simulink model "UnusedModels"  (R2015a)
settings: Solver=ode45  StartTime=0.0  StopTime=10.0  RelTol=1e-3
values from neighbouring files (symbols this model uses):
  car_params = Simulink_Car_params    [TV2016_parameters.m]
  energyLimitControl = Simulink_energyLimit    [TV2016_parameters.m]
  settings = Simulink_Settings    [TV2016_parameters.m]
  speedEstimation = Simulink_speedEst    [TV2016_parameters.m]
  tractionControl = Simulink_tc    [TV2016_parameters.m]
  yawRateControl = Simulink_yawRate    [TV2016_parameters.m]
undefined symbols (not defined in the file or in its folder): canChannel, Use_Estimated_velocity
libraries: canlib x44, CarMaker4SL x33, canmsglib x28, simulink x6
(part 3 of 4)

== matlab function UnusedModels/speedEstimate/Vestimate ==
  data: sensors input; V_est_x output; whl_speed output Bus: Whl_speed; Y_meas output; front_rear_Var output; front_Var output; rear_Var output; all_Var output; left_Var output; right_Var output; RPM_derivative input Bus: RPMDerivative; normalForces input Bus: normalForces; settings parameter; car_params parameter; speedEstimation parameter
function [V_est_x,whl_speed, Y_meas,front_rear_Var,front_Var,rear_Var,all_Var,left_Var,right_Var]...
         = SpeedEstimations(sensors,RPM_derivative,normalForces,settings,car_params,speedEstimation)
     
     
     %rateRPM_FL, rateRPM_FR,rateRPM_RL,rateRPM_RR,sensor,settings,car_params)
%#codegen

% ------------------------------
% DECLARATIONS
% ------------------------------
persistent firstIteration;
persistent v;
persistent error;
persistent K;
k_FL = single(0); % Gain 
k_FR = single(0); % Gain
k_RL = single(0); % Gain
k_RR = single(0); % Gain
% Gains for trusting, not trusting wheel speed measurements
Hg = speedEstimation.High_gain;
Lg = speedEstimation.Low_gain;
% Variances
all_Var = single(0); % Variance for all measurements
front_rear_Var = single(0);
front_Var = single(0);
rear_Var = single(0);
left_Var = single(0);
right_Var = single(0);
% LIMITS:
velocity_deviation_limit = speedEstimation.velocity_deviation_limit;
lim = speedEstimation.variance_limit;
RPM_derivative_limit = speedEstimation.RPM_derivative_limit;

% Measurement vector
C = [1;1;1;1]; % Create four copies of predicted vx

pikk = int32(50);
% ------------------------------
% PARAMETERS
% ------------------------------
%Conversion from RPM to rad/s for the wheel
c = single(2*pi/(car_params.GR*60));
t = settings.control_system_sample_time;
%Weights taken from wikipedia
%sg_Weight = single( [ 1; -8; 0; 8; -1] );
sg_Weight = single( [ -1; 8; 0; -8; 1] );
%sg_Weight = single([0.3; 0.1; -0.1 ; -0.3]);
%sg_Weight = single([1; -1; 0 ; -0]);
% ------------------------------
% COPY VARIABLES EACH TIMESTEP
% ------------------------------
S = sensors.Input_steering; % Steering angle in rad( Mean of front wheels)
ax = sensors.ax; % Should be true linear acceleration compensated for roll angle
%Fz, used to determine what wheel speeds to trust.
Fz = [normalForces.FL, normalForces.FR, normalForces.RL ,normalForces.RR];
% Determine CoG Vx from motor RPM. Simple atm. Not considering vy.
Whl_v_FL = sensors.RPM_FL*c*car_params.r_eff*cos(S) + sensors.r*car_params.t_f;
Whl_v_FR = sensors.RPM_FR*c*car_params.r_eff*cos(S) - sensors.r*car_params.t_f;
Whl_v_RL = sensors.RPM_RL*c*car_params.r_eff + sensors.r*car_params.t_r;
Whl_v_RR = sensors.RPM_RR*c*car_params.r_eff - sensors.r*car_params.t_r;
whl_speed.v_FL = Whl_v_FL;
whl_speed.v_FR = Whl_v_FR;
whl_speed.v_RL = Whl_v_RL;
whl_speed.v_RR = Whl_v_RR;


RPM = [sensors.RPM_FL, sensors.RPM_FR, sensors.RPM_RL, sensors.RPM_RR]';
% Measurement vector, compensated RPMS
Y_meas = [Whl_v_FL, Whl_v_FR, Whl_v_RL, Whl_v_RR]';
% Input Derivative of RPM
rateRPM_FL = RPM_derivative.FL;
rateRPM_FR = RPM_derivative.FR;
rateRPM_RL = RPM_derivative.RL;
rateRPM_RR = RPM_derivative.RR;

% Different sums of normal forces, used to determine what wheels to trust
left_Fz = sum(Fz([1 3]));
right_Fz = sum(Fz([2 4]));
front_Fz = sum(Fz(1:2));
rear_Fz = sum(Fz(3:4));

% ------------------------------
% ESTIMATE DERIVATIVE OF COMPENSATED MOTOR RPM
% ------------------------------
% Problem with noise from yaw rate coupling into the derivative.. 
% Can I use uncompensated front wheels ? Should not be slipping like crazy
% with a significant steering angle ? 

% First try is with pure RPMS
% rateRPM_FL = simpleNumericalDerivative_RPM(sensor.RPM_FL,t);
% rateRPM_FR = simpleNumericalDerivative_RPM(sensor.RPM_FR,t);
% rateRPM_RL = simpleNumericalDerivative_RPM(sensor.RPM_RL,t);
% rateRPM_RR = simpleNumericalDerivative_RPM(sensor.RPM_RR,t);


% ------------------------------
% DRIFTING INS VELOCITY
% ------------------------------
persistent drift;




% ALGORITHM
if isempty(firstIteration)
    K = single(ones(1,4));
    v = single(0);
    V_est_x = v;
    error = Y_meas- C*v;
    firstIteration = 2;
    drift = single(0);
else
    drift = drift + 0.03*t;
    v_ins = sensors.V_x + 0.05 + drift;
    v = v + t*ax;
    %v = v + t*(ax + K*error);
    error = Y_meas - C*v ;
    V_est_x = 0.98*v;
    
    % Find K
    % Divide by zero problems...
    mean_WhlV = max(0.001,mean(Y_meas));
    mean_front_WhlV = max(0.001,mean(Y_meas(1:2)));
    mean_rear_WhlV  = max(0.001,mean(Y_meas(3:4)));
    mean_left_WhlV  = max(0.001,mean(Y_meas([1 3])));
    mean_right_WhlV = max(0.001,mean(Y_meas([2 4])));

    all_Var = var(Y_meas,1)/mean_WhlV;
    front_rear_Var = var([mean_front_WhlV, mean_rear_WhlV],1)/mean_WhlV;
    front_Var = var(Y_meas(1:2),1)/mean_front_WhlV;
    rear_Var  = var(Y_meas(3:4),1)/mean_rear_WhlV;
    
    left_Var    = var(Y_meas([1 3]),1)/mean_left_WhlV;
    right_Var   = var(Y_meas([2 4]),1)/mean_right_WhlV;   
    
    if (  (abs(Whl_v_FL - v_ins) > velocity_deviation_limit)...
       && (abs(Whl_v_FR - v_ins) > velocity_deviation_limit)...
       && (abs(Whl_v_RL - v_ins) > velocity_deviation_limit)...
       && (abs(Whl_v_RR - v_ins) > velocity_deviation_limit) )
        
        K = [Lg, Lg, Lg, Lg];
    
    elseif (all_Var  < lim ) 
        % low variance for all wheels.
        % Check derivative of motor RPM
        if ( (rateRPM_FL > RPM_derivative_limit) ||...
             (rateRPM_FR > RPM_derivative_limit) ||...
             (rateRPM_RL > RPM_derivative_limit) ||...
             (rateRPM_RR > RPM_derivative_limit))
            K = [Lg, Lg, Lg, Lg];
        % Rate of change of RPM can be low but slip rate is large
        % Check against drifting INS velocity 
        else
            K = [Hg, Hg ,Hg ,Hg];
        end
    % Variance is high. What wheel(s) are causing this.. 
    % STRUCTURE:
    % 1 = FRONT AND REAR DIFFER
    % 2 = LEFT AND RIGHT DIFFER
    % 3 = FL WRONG
    % 4 = FR WRONG
    % 5 = RL WRONG
    % 6 = RR WRONG
    % 7 Combinations of 3-6 that are not handled in 1-2.
    
    %1: FRONT AND REAR DIFFER
    elseif( (right_Var > front_Var) && (right_Var > rear_Var)...
            && (left_Var > front_Var) && (left_Var > rear_Var))
        % High variance between front and rear, and low variance 
        % at front and rear.
        
        % Also need to check if front/rear wheels are slipping
        
        % Front wheels over limit while rear is ok
        if (((rateRPM_FL > RPM_derivative_limit) ||...
             (rateRPM_FR > RPM_derivative_limit)) &&...
            ((rateRPM_RL < RPM_derivative_limit) ||...
             (rateRPM_RR < RPM_derivative_limit)) )
             
            K = [Lg, Lg, Hg, Hg];
        % Rear wheels over limit while front is ok
        elseif ( ((rateRPM_FL < RPM_derivative_limit) ||...
                 (rateRPM_FR < RPM_derivative_limit)) &&...
                ((rateRPM_RL > RPM_derivative_limit) ||...
                 (rateRPM_RR > RPM_derivative_limit)) )
             K = [Hg, Hg, Lg, Lg];
        % All are over limit
        elseif  ((rateRPM_FL > RPM_derivative_limit) &&...
                 (rateRPM_FR > RPM_derivative_limit) &&...
                 (rateRPM_RL > RPM_derivative_limit) &&...
                 (rateRPM_RR > RPM_derivative_limit) ) 
              K = [Lg, Lg, Lg, Lg];
              
        % The rate of change of RPM will flatten out and the high
        % slip ratio will still exist. Handle this
        
        % Check big difference in wheel speeds
        % Two cases. Driving and braking. 
        
        % Driving. Need logic to determine driving/braking
        elseif ( (RPM(1) + RPM(2)) > (RPM(3) + RPM(4)) )
            K = [Lg, Lg, Hg, Hg];
        elseif ( (RPM(1) + RPM(2)) < (RPM(3) + RPM(4)) )
            K = [Hg, Hg, Lg, Lg];
            % If frontFZ - rearFZ < 0, then FL is set to 0
            % Else it is set to a positive gain
%             k_FL = (1/abs(front_Fz-rear_Fz))*max(0,front_Fz - rear_Fz);
%             k_FR = (1/abs(front_Fz-rear_Fz))*max(0,front_Fz - rear_Fz);
% 
%             k_RL = (1/abs(rear_Fz-front_Fz))*max(0,rear_Fz-front_Fz)*0.5;
%             k_RR = (1/abs(rear_Fz-front_Fz))*max(0,rear_Fz-front_Fz)*0.5;
%            K = [k_FL, k_FR, k_RL, k_RR];
        end
    %2: LEFT AND RIGHT WHEELS DIFFER
    elseif ( ((front_Var > right_Var) && (rear_Var > right_Var)) ||...
            ( (front_Var > left_Var) && (rear_Var > left_Var)))
   
        k_FL = (1/abs(left_Fz-right_Fz))*max(0,left_Fz - right_Fz);
        k_RL = (1/abs(left_Fz-right_Fz))*max(0,left_Fz - right_Fz);
        
        k_FR = (1/abs(right_Fz-left_Fz))*max(0,right_Fz-left_Fz);
        k_RR = (1/abs(right_Fz-left_Fz))*max(0,right_Fz-left_Fz);
        
        K = [k_FL, k_FR, k_RL, k_RR];
        
    %3: FL WRONG
    elseif ( (left_Var > rear_Var) && (left_Var > right_Var)...
            && (front_Var > rear_Var) )
        k_FL = single(0);
        k_FR = single(0);
        k_RL = single(1);
        k_RR = single(1);
        K = [k_FL, k_FR, k_RL, k_RR];
    %4: FR WRONG
    elseif ( (right_Var > rear_Var) && (right_Var > left_Var)...
            && (front_Var > rear_Var))
        k_FL = single(0);
        k_FR = single(0);
        k_RL = single(1);
        k_RR = single(1);
        K = [k_FL, k_FR, k_RL, k_RR]; 
    %5: RL WRONG
    elseif ( (left_Var > front_Var) && (left_Var > right_Var)...
            && (rear_Var > front_Var))
        
        k_FL = single(1);
        k_FR = single(1);
        k_RL = single(0);
        k_RR = single(0);
        K = [k_FL, k_FR, k_RL, k_RR]; 
        
    %5: RR WRONG    
    elseif ( (right_Var > front_Var) && (right_Var > left_Var)...
            && (rear_Var > front_Var))
        k_FL = single(1);
        k_FR = single(1);
        k_RL = single(0);
        k_RR = single(0);
        K = [k_FL, k_FR, k_RL, k_RR]; 
    else
        k_FL = single(0);
        k_FR = single(0);
        k_RL = single(0);
        k_RR = single(0);
        K = [k_FL, k_FR, k_RL, k_RR]; 
    end
   
end
end

% function rateRPM = simpleNumericalDerivative_RPM(RPM, ts)
%     persistent firstIteration;
%     persistent RPM_prev;
%     
%     if isempty(firstIteration)
%         firstIteration = 2;
%         RPM_prev = RPM;
%         rateRPM = single(0);
%     else
%         %Calculate output
%         rateRPM = abs( (RPM - RPM_prev)/(ts));
%         RPM_prev = RPM;
%         if (rateRPM > 1000000)
%             rateRPM = single(0);
%         end
%     end    
% end



% function rateRPM = savitzkyGolay_RPM(RPM,nr_Coefficients,weight_Vector,ts)
%     % y(k) is rate of change of input variable per time step (ts) 
%     % means divide y(k) by ts 
%     % RPM is 4x1
%     % Weight vector is 4x1
%     persistent firstIteration;
%     persistent frame;
%  
%     % Filter at midpoint of dataset
%     % Assume even filter coeffs
%     midPoint = uint32(nr_Coefficients);
%     
%     % Declare
%     
%     rateRPM = single(0);
% 
%     if isempty(firstIteration)
%         firstIteration = 2;
%         frame = single(zeros(1,nr_Coefficients));
%         rateRPM = single(0);
%     else
%         %Update frame
%         % Newest first, discard last element
%         frame = [RPM, frame(1:(end-1))]
%         
%         %Calculate output
%         rateRPM = abs((frame*weight_Vector)./(12*ts));
%         if (rateRPM > 400000)
%             rateRPM = single(0);
%         end
%         
%     end
% end


%     
% double sg_filter(const double raw_data[5])
% {
%     const int i = 2;
%     double result(0);
%     
%     result = (1.0/35.0) * ( - 3.0*raw_data[i-2]  
%                             + 12.0*raw_data[i-1]
%                             + 17.0*raw_data[i]  
%                             + 12.0*raw_data[i+1] 
%                             - 3.0*raw_data[i+2] );
%     return result;
% }
%         
%     
%     

        
    
        
        



            
    %ONE WHEEL AT FRONT AND ONE AT REAR IS INACCURATE.
    % If Fz left > Fz right AND left_Var < limit  -> trust left wheels
    % If Fz right < Fz right AND right_Var < limit -> trust right wheels
    
    %TWO WHEELS AT EITHER FRONT OR REAR ARE WRONG
    
    
    %
        
    % Find Gains in K
    % Hvis alle er ca samme, høy gain
    % Hvis front/rear left/right er forskjellige, stol på de to med mest
    % normalkrefter 
    
    % Essensen er: Hvis fysiske conditions tilsier at hjulfart = bilfart,
    % sett høy Ki. 
    
    % Variansen av et sett med målinger for ett hjul ? 
    
    % Ta covariansen for ax run?
    % Covariance for skidpad run?
    
    
    % If all wheels are approx the same, I still need to check for 
    % physical stuff, such as how fast the rpm is increasing.
    
    %Acceleration:
    %All wheels can slip hence max rate of change is valid 
   
    %Skidpad:
    %All wheels can slip at start
    %If negative torque, braking slip can occur.. 
    
    
    % If front / rear are pretty equal, then since variance of all is
    % pretty high. Must imply that either F_LR or R_LR, or (F_LR && R_LR)
    % is high.
    
    % One wheel is spinning ( FL) , total var is high, FR var > limit
    % -> low var rear , high var front. trust only rear wheels.

== matlab function UnusedModels/Allocates Torque. Engineering solution1 ==
  data: Ti_lim output Bus: Ti_lim; T_req input; states input; settings parameter; car_params parameter; Mz_ref input; Ti_max output; Mz_error output; Mz_allocated output; yawRateControl parameter
function [Ti_lim,Ti_max,Mz_error, Mz_allocated]  = torqueAllocation(T_req,states,settings, car_params, Mz_ref,yawRateControl)
%#codegen
%STATES
r = states.r;

%PARAMETERS
mu = settings.mui;
tf = car_params.t_f*2;
tr = car_params.t_r*2;
GR = car_params.GR;
r_eff = car_params.r_eff;
R = [r_eff; r_eff; r_eff; r_eff]';
%Load Transfer
Fzi = [states.Fz_FL states.Fz_FR states.Fz_RL states.Fz_RR]';
alfa_r =  (Fzi(3) + Fzi(4)) / (Fzi(1) + Fzi(2) + Fzi(3) + Fzi(4));
%MZ
S = states.steering_angle;
% l1 = car_params.t_f*cos(S) - car_params.l_f*sin(S); 
% l2 = car_params.t_f*cos(S) + car_params.l_f*sin(S);

l1 = car_params.t_f*cos(S);
l2 = car_params.t_f*cos(S);
l3 = car_params.t_r;
l4 = car_params.t_r;
L = [-l1; l2; -l3; l4];

%FIND MAXIMUM ALLOWED MOTOR TORQUE, TIRE/MOTOR
Ti_max          = single(zeros(4,1));
Ti_max_tire     = single(zeros(4,1));
Ti_max_motor    = single(zeros(4,1));

RPM = [states.RPM_FL, states.RPM_FR, states.RPM_RL, states.RPM_RR];
a = 8/7000;
a2 = 13/1000;
for i=1:4
    if RPM(i) >= 20000 
        Ti_max_motor(i) = 0;
    elseif RPM(i) > 12000 & RPM(i) < 19000
        Ti_max_motor(i) = -a*(RPM(i) - 12000) + 21;
    elseif RPM(i) > 19000 & RPM(i) < 20000
        Ti_max_motor(i) = -a2*(RPM(i) - 19000) + 13;
    else 
        Ti_max_motor(i) = settings.max_motor_torque;
    end
end


%Tire saturation based on mu and Fz
for i=1:4
    Ti_max_tire(i) = Fzi(i)*mu*R(i)/GR;
end
% Find minimum of tire saturation Torque and motor
for i=1:4
    Ti_max(i) = min(Ti_max_tire(i), Ti_max_motor(i));
end
%**********************************************%

T_F = single(zeros(2,1));
T_R = single(zeros(2,1));
sat_F = uint32(0);
sat_R = uint32(0);


front_sat = 0;
rear_sat = 0;
if ( T_req >= 0)
    [T_F, sat_F] = torqueVectoring(Ti_max(1), Ti_max(2), T_req, R(1), R(2), (1-alfa_r), Mz_ref, GR, tf,Fzi(1), Fzi(2));
    [T_R, sat_R] = torqueVectoring(Ti_max(3), Ti_max(4), T_req, R(3), R(4), alfa_r, Mz_ref, GR, tr, Fzi(3), Fzi(4));
    if ( (sat_F == 1) && (sat_R == 1) )
        % Nothing more to do
    elseif ( (sat_F == 1) && (sat_R == 0) )    
         front_sat = 1;
         if ( T_F(1) < 0) 
            T_remaining = T_req - (T_F(2));
         elseif (T_F(2) < 0) 
             T_remaining = T_req - (T_F(1));
         else
             T_remaining = T_req - (T_F(1) + T_F(2));
         end
         
         %T_remaining = T_req - (T_F(1) + T_F(2));
         %Mz_remaining = Mz_ref*alfa_r;
         
         if (yawRateControl.enable == 1)
             Mz_remaining = Mz_ref - (-l1*GR*T_F(1)/R(1) + l2*GR*T_F(2)/R(2));
         else
             Mz_remaining = single(0);
         end 
         [T_R sat_R] = torqueVectoring(Ti_max(3), Ti_max(4), T_remaining, R(3), R(4), 1 , Mz_remaining, GR, tr, Fzi(3), Fzi(4));
    elseif ( (sat_F == 0) && (sat_R == 1) )
        rear_sat = 1;
         if ( T_R(1) < 0) 
            T_remaining = T_req - (T_R(2));
         elseif (T_R(2) < 0) 
             T_remaining = T_req - (T_R(1));
         else
             T_remaining = T_req - (T_R(1) + T_R(2));
         end        
        % For example rear is saturated, and front can still use more torque
        %T_remaining = T_req - (T_R(1) + T_R(2));
        if (yawRateControl.enable == 1)
             Mz_remaining = Mz_ref - (-l3*GR*T_R(1)/R(3) + l4*GR*T_R(2)/R(4));
        else
             Mz_remaining = single(0);
        end 
        %Mz_remaining = Mz_ref*(1-alfa_r);
        [T_F sat_F] = torqueVectoring(Ti_max(1), Ti_max(2), T_remaining, R(1), R(2), 1 , Mz_remaining, GR, tf, Fzi(1), Fzi(2)); 
    else
        %both false
        % Nothing to do here either
    end
else
    %Negative torque
    [T_F, sat_F] = allocateNegativeTorque(Ti_max(1), Ti_max(2), T_req, R(1), R(2), (1-alfa_r), Mz_ref, GR, tf,Fzi(1), Fzi(2));
    [T_R, sat_R] = allocateNegativeTorque(Ti_max(3), Ti_max(4), T_req, R(3), R(4), alfa_r, Mz_ref, GR, tr, Fzi(3), Fzi(4));
    if (sat_F == 1 && sat_R == 1)
        %Nothing more to do
    elseif (sat_F == 1 && sat_R == 0)
         T_remaining = T_req - (T_F(1) + T_F(2));
         %Disable Mz_remaining if yaw control disabled?
        if (yawRateControl.enable == 1)
             Mz_remaining = Mz_ref - (-l1*GR*T_F(1)/R(1) + l2*GR*T_F(2)/R(2));
        else
             Mz_remaining = single(0);
        end
         %Mz_remaining = Mz_ref*alfa_r;
         [T_R sat_R] = allocateNegativeTorque(Ti_max(3), Ti_max(4), T_remaining, R(3), R(4), 1 , Mz_remaining, GR, tr, Fzi(3), Fzi(4));
    elseif (sat_F == 0 && sat_R == 1)
        %For example rear is saturated, and front can still use more torque
        T_remaining = T_req - (T_R(1) + T_R(2));
        %Mz_remaining = Mz_ref*(1-alfa_r);
        
        if (yawRateControl.enable == 1)
             Mz_remaining = Mz_ref - (-l3*GR*T_R(1)/R(3) + l4*GR*T_R(2)/R(4));
        else
             Mz_remaining = single(0);
        end
        [T_F sat_F] = allocateNegativeTorque(Ti_max(1), Ti_max(2), T_remaining, R(1), R(2), 1 , Mz_remaining, GR, tf, Fzi(1), Fzi(2)); 
    else
        %both false
        %Nothing to do here either
    end
end

Ti_all = [T_F' T_R'];

Ti_lim_struct = struct;
Ti_lim_struct.FL = Ti_all(1);
Ti_lim_struct.FR = Ti_all(2);
Ti_lim_struct.RL = Ti_all(3);
Ti_lim_struct.RR = Ti_all(4);

Ti_lim = Ti_lim_struct;

% Calculate what yaw moment that was achieved with the current 
% allocation
Fx_all = prod([Ti_all; 1./R;])*GR;
Mz_allocated = L'*Fx_all';
Mz_error = Mz_ref - Mz_allocated;

end

function [T, sat] = torqueVectoring(L_max, R_max, T_req,...
          R_eff_L, R_eff_R, alfa, Mz_ref, GR, t, Fz_L,Fz_R )
      
    T = single(zeros(2,1));
    sat = uint32(0);
    % Desired torque vectoring torque
    TV_des = abs(alfa*Mz_ref*R_eff_L/(GR*t)) + abs(alfa*Mz_ref*R_eff_R/(GR*t));
    % Take absolute value since T_req can be negative in case of KERS
    T_driver = alfa*T_req;

    if ( Mz_ref <= 0)
        % Implies that left side should realize the TV torque,
        % since only torque >= 0 is used here.
        % Mz is defined positive counter clockwise
        L = min( [TV_des, T_driver, L_max]);
        %Max torque that can be added to both
        if ( (L + 0.0001) < abs(TV_des))
            % Add negative torque...
            R = -min( (TV_des-L), R_max);
            if ( (L + 0.001) < (T_driver))
                sat = uint32(1);
            end
            T = [L;R];
            return
        else          
            max_t_add = min([(L_max-TV_des), R_max, (T_driver-L)/2]);
            R = max_t_add;
            L = L + max_t_add;
            if ( (L + R + 0.001) < (T_driver))
                sat = uint32(1);
            end
            T = [L;R];
            return
        end 
    else
        R = min( [abs(TV_des), T_driver, R_max]);
        %Max torque that can be added to both
        if ( (R + 0.0001) < abs(TV_des))
            % Add negative torque...
            L = -min( (TV_des-R), L_max);
            if ( (R + 0.001) < (T_driver))
                sat = uint32(1);
            end
            T = [L;R];
            return
        else
            max_t_add = min([(R_max-TV_des), L_max, (T_driver-R)/2]);
            R = R + max_t_add;
            L = max_t_add;
            if ( (L + R + 0.001) < (T_driver))
                sat = uint32(1);
            end 
            T = [L;R];
            return                 
        end
    end
end

function [T, sat] = allocatePositiveTorque(L_max, R_max, T_req,...
          R_eff_L, R_eff_R, alfa, Mz_ref, GR, t, Fz_L,Fz_R )
      
    T = single(zeros(2,1));
    sat = uint32(0);
    % Desired torque vectoring torque
    TV_des = abs(alfa*Mz_ref*R_eff_L/(GR*t)) + abs(alfa*Mz_ref*R_eff_R/(GR*t));
    % Take absolute value since T_req can be negative in case of KERS
    T_driver = alfa*T_req;

    if ( Mz_ref <= 0)
        % Implies that left side should realize the TV torque,
        % since only torque >= 0 is used here.
        % Mz is defined positive counter clockwise
        L = min( [TV_des, T_driver, L_max]);
        %Max torque that can be added to both
        if L_max < abs(TV_des)
            max_t_add = single(0);
        else
            max_t_add = min([(L_max-TV_des), R_max, (T_driver-L)/2]);
        end 
        L = L + max_t_add;
        R = max_t_add;
        T = [L;R];  
        % Floats comparison
        if ( (L + R + 0.001) < (T_driver))
            sat = uint32(1);
        end
        return;
    else
        R = min( [abs(TV_des), T_driver, R_max]);
        %Max torque that can be added to both
        if R_max < abs(TV_des)
            max_t_add = single(0);
        else
            max_t_add = min([(R_max-abs(TV_des)),L_max, (T_driver-R)/2]);
        end
        R = R + max_t_add;
        L = max_t_add;
        T = [L;R];
        % Floats comparison
        if ( (L + R + 0.001) < (T_driver))
            sat = uint32(1);
        end
        return;
    end
end

function [T, sat] = allocateNegativeTorque(L_max, R_max, T_req, R_eff_L, R_eff_R, alfa, Mz_ref, GR, t, Fz_L,Fz_R )
    T = single(zeros(2,1));
    sat = uint32(0);
    % Desired torque vectoring torque
    TV_des = abs(alfa*Mz_ref*R_eff_L/(GR*t)) + abs(alfa*Mz_ref*R_eff_R/(GR*t));
    % Take absolute value since T_req can be negative in case of KERS
    T_driver = abs(alfa*T_req);
   
    if (Mz_ref + 0.0001 >= 0)
        % Positive Mz_ref requires left side (inner wheels)
        % to brake more than the outer wheels.
        L = min( [TV_des, T_driver, L_max]);
        %Max torque that can be added to both
        if L_max < abs(TV_des)
            max_t_add = single(0);
        else
            max_t_add = min([(L_max-TV_des), R_max, (T_driver-L)/2]);
        end 
        L = - (L + max_t_add);
        R = - max_t_add;
        T = [L;R];
        % Floats comparison
        if ( (abs(L) + abs(R) + 0.001) < T_driver)
            sat = uint32(1);
        end
        return;
    else
        R = min( [abs(TV_des), T_driver, R_max]);
        %Max torque that can be added to both
        if R_max < abs(TV_des)
            max_t_add = single(0);
        else
            max_t_add = min([(R_max-abs(TV_des)),L_max, (T_driver-R)/2]);
        end
        R = - (R + max_t_add);
        L = - max_t_add;
        T = [L;R];
        % Floats comparison
        if ( (abs(L) + abs(R) + 0.001) < T_driver)
            sat = uint32(1);
        end
        return;
    end
end


function [T, sat] = distOuter(L_max, R_max, T_req,...
    R_eff_L, R_eff_R, alfa, Mz_ref, GR, t, Fz_L,Fz_R )
    T = single(zeros(2,1));
    sat = uint32(0);
    % Desired torque vectoring torque
    TV_des = abs(alfa*Mz_ref*R_eff_L/(GR*t)) +...
            abs(alfa*Mz_ref*R_eff_R/(GR*t));
    % Take absolute value since T_req can be negative in case of KERS
    T_driver = abs(alfa*T_req);   
    if Fz_L >= Fz_R
        % Implies that left side should realize the TV torque
        L = min( [TV_des, T_driver, L_max]);
        %Max torque that can be added to both
        if L_max < abs(TV_des)
            max_t_add = single(0);
        else
            max_t_add = min([(L_max-TV_des), R_max, (T_driver-L)/2]);
        end 
        L = L + max_t_add;
        R = max_t_add;
        T = [L;R];
        if ( (L + R) < T_driver)
            sat = uint32(1);
        end
        return;
    elseif Fz_L < Fz_R
        R = min( [abs(TV_des), T_driver, R_max]);
        %Max torque that can be added to both
        if R_max < abs(TV_des)
            max_t_add = single(0);
        else
            max_t_add = min([(R_max-abs(TV_des)),L_max, (T_driver-R)/2]);
        end
        R = R + max_t_add;
        L = max_t_add;
        T = [L;R];
        if ( (L + R) < T_driver)
            sat = uint32(1);
        end
        return;
    end
end

== matlab function UnusedModels/Allocates Torque. Engineering solution ==
  data: Ti_lim output Bus: Ti_lim; T_req input; states input; settings parameter; car_params parameter; Mz_ref input; Ti_max output; Mz_error output; front_sat output; rear_sat output; yawRateControl parameter
function [Ti_lim,Ti_max,Mz_error, front_sat,rear_sat]  = torqueAllocation(T_req,states,settings, car_params, Mz_ref,yawRateControl)
%#codegen
%STATES
r = states.r;

%PARAMETERS
mu = settings.mui;
tf = car_params.t_f*2;
tr = car_params.t_r*2;
GR = car_params.GR;
r_eff = car_params.r_eff;
R = [r_eff; r_eff; r_eff; r_eff]';
%Load Transfer
Fzi = [states.Fz_FL states.Fz_FR states.Fz_RL states.Fz_RR]';
alfa_r =  (Fzi(3) + Fzi(4)) / (Fzi(1) + Fzi(2) + Fzi(3) + Fzi(4));
%MZ
S = states.steering_angle;
l1 = car_params.t_f*cos(S) - car_params.l_f*sin(S); 
l2 = car_params.t_f*cos(S) + car_params.l_f*sin(S);
l3 = car_params.t_r;
l4 = car_params.t_r;
L = [-l1; l2; -l3; l4];

%FIND MAXIMUM ALLOWED MOTOR TORQUE, TIRE/MOTOR
Ti_max          = single(zeros(4,1));
Ti_max_tire     = single(zeros(4,1));
Ti_max_motor    = single(zeros(4,1));

RPM = [states.RPM_FL, states.RPM_FR, states.RPM_RL, states.RPM_RR];
a = 8/7000;
a2 = 13/1000;
for i=1:4
    if RPM(i) >= 20000 
        Ti_max_motor(i) = 0;
    elseif RPM(i) > 12000 & RPM(i) < 19000
        Ti_max_motor(i) = -a*(RPM(i) - 12000) + 21;
    elseif RPM(i) > 19000 & RPM(i) < 20000
        Ti_max_motor(i) = -a2*(RPM(i) - 19000) + 13;
    else 
        Ti_max_motor(i) = settings.max_motor_torque;
    end
end


%Tire saturation based on mu and Fz
for i=1:4
    Ti_max_tire(i) = Fzi(i)*mu*R(i)/GR;
end
% Find minimum of tire saturation Torque and motor
for i=1:4
    Ti_max(i) = min(Ti_max_tire(i), Ti_max_motor(i));
end
%**********************************************%

T_F = single(zeros(2,1));
T_R = single(zeros(2,1));
sat_F = uint32(0);
sat_R = uint32(0);


front_sat = 0;
rear_sat = 0;
if ( T_req >= 0)
    [T_F, sat_F] = allocatePositiveTorque(Ti_max(1), Ti_max(2), T_req, R(1), R(2), (1-alfa_r), Mz_ref, GR, tf,Fzi(1), Fzi(2));
    [T_R, sat_R] = allocatePositiveTorque(Ti_max(3), Ti_max(4), T_req, R(3), R(4), alfa_r, Mz_ref, GR, tr, Fzi(3), Fzi(4));
    [T_F, sat_F] = negative(Ti_max(1), Ti_max(2), T_req, R(1), R(2), (1-alfa_r), Mz_ref, GR, tf,Fzi(1), Fzi(2));
    [T_R, sat_R] = allocatePositiveTorque(Ti_max(3), Ti_max(4), T_req, R(3), R(4), alfa_r, Mz_ref, GR, tr, Fzi(3), Fzi(4));    

    if ( (sat_F == 1) && (sat_R == 1) )
        % Nothing more to do
    elseif ( (sat_F == 1) && (sat_R == 0) )    
         front_sat = 1;
         T_remaining = T_req - (T_F(1) + T_F(2));
         %Mz_remaining = Mz_ref*alfa_r;
         
         if (yawRateControl.enable == 1)
             Mz_remaining = Mz_ref - (-l1*GR*T_F(1)/R(1) + l2*GR*T_F(2)/R(2));
         else
             Mz_remaining = single(0);
         end 
         [T_R sat_R] = allocatePositiveTorque(Ti_max(3), Ti_max(4), T_remaining, R(3), R(4), 1 , Mz_remaining, GR, tr, Fzi(3), Fzi(4));
    elseif ( (sat_F == 0) && (sat_R == 1) )
        rear_sat = 1;
        % For example rear is saturated, and front can still use more torque
        T_remaining = T_req - (T_R(1) + T_R(2));
        if (yawRateControl.enable == 1)
             Mz_remaining = Mz_ref - (-l3*GR*T_R(1)/R(3) + l4*GR*T_R(2)/R(4));
        else
             Mz_remaining = single(0);
        end 
        %Mz_remaining = Mz_ref*(1-alfa_r);
        [T_F sat_F] = allocatePositiveTorque(Ti_max(1), Ti_max(2), T_remaining, R(1), R(2), 1 , Mz_remaining, GR, tf, Fzi(1), Fzi(2)); 
    else
        %both false
        % Nothing to do here either
    end
else
    %Negative torque
    [T_F, sat_F] = allocateNegativeTorque(Ti_max(1), Ti_max(2), T_req, R(1), R(2), (1-alfa_r), Mz_ref, GR, tf,Fzi(1), Fzi(2));
    [T_R, sat_R] = allocateNegativeTorque(Ti_max(3), Ti_max(4), T_req, R(3), R(4), alfa_r, Mz_ref, GR, tr, Fzi(3), Fzi(4));
    if (sat_F == 1 && sat_R == 1)
        %Nothing more to do
    elseif (sat_F == 1 && sat_R == 0)
         T_remaining = T_req - (T_F(1) + T_F(2));
         %Disable Mz_remaining if yaw control disabled?
        if (yawRateControl.enable == 1)
             Mz_remaining = Mz_ref - (-l1*GR*T_F(1)/R(1) + l2*GR*T_F(2)/R(2));
        else
             Mz_remaining = single(0);
        end
         %Mz_remaining = Mz_ref*alfa_r;
         [T_R sat_R] = allocateNegativeTorque(Ti_max(3), Ti_max(4), T_remaining, R(3), R(4), 1 , Mz_remaining, GR, tr, Fzi(3), Fzi(4));
    elseif (sat_F == 0 && sat_R == 1)
        %For example rear is saturated, and front can still use more torque
        T_remaining = T_req - (T_R(1) + T_R(2));
        %Mz_remaining = Mz_ref*(1-alfa_r);
        
        if (yawRateControl.enable == 1)
             Mz_remaining = Mz_ref - (-l3*GR*T_R(1)/R(3) + l4*GR*T_R(2)/R(4));
        else
             Mz_remaining = single(0);
        end
        [T_F sat_F] = allocateNegativeTorque(Ti_max(1), Ti_max(2), T_remaining, R(1), R(2), 1 , Mz_remaining, GR, tf, Fzi(1), Fzi(2)); 
    else
        %both false
        %Nothing to do here either
    end
end

Ti_all = [T_F' T_R'];

Ti_lim_struct = struct;
Ti_lim_struct.FL = Ti_all(1);
Ti_lim_struct.FR = Ti_all(2);
Ti_lim_struct.RL = Ti_all(3);
Ti_lim_struct.RR = Ti_all(4);

Ti_lim = Ti_lim_struct;

% Calculate what yaw moment that was achieved with the current 
% allocation
Fx_all = prod([Ti_all; 1./R;])*GR;
Mz_allocated = L'*Fx_all';
Mz_error = Mz_ref - Mz_allocated;

end

function [T, sat] = negative(L_max, R_max, T_req,...
          R_eff_L, R_eff_R, alfa, Mz_ref, GR, t, Fz_L,Fz_R )
      
    T = single(zeros(2,1));
    sat = uint32(0);
    % Desired torque vectoring torque
    TV_des = abs(alfa*Mz_ref*R_eff_L/(GR*t)) + abs(alfa*Mz_ref*R_eff_R/(GR*t));
    % Take absolute value since T_req can be negative in case of KERS
    T_driver = alfa*T_req;

    if ( Mz_ref <= 0)
        % Implies that left side should realize the TV torque,
        % since only torque >= 0 is used here.
        % Mz is defined positive counter clockwise
        L = min( [TV_des, T_driver, L_max]);
        %Max torque that can be added to both
        if L < abs(TV_des)
            % Add negative torque...
            R = -min( (TV_des-L), R_max);
            if ( (L + 0.001) < (T_driver))
                sat = uint32(1);
            end
            T = [L;R];
            return
        else          
            max_t_add = min([(L_max-TV_des), R_max, (T_driver-L)/2]);
            R = max_t_add;
            L = L + max_t_add;
            if ( (L + R + 0.001) < (T_driver))
                sat = uint32(1);
            end
            T = [L;R];
            return
        end 
    else
        R = min( [abs(TV_des), T_driver, R_max]);
        %Max torque that can be added to both
        if R < abs(TV_des)
            % Add negative torque...
            L = -min( (TV_des-R), L_max);
            if ( (R + 0.001) < (T_driver))
                sat = uint32(1);
            end
            T = [L;R];
            return
        else
            max_t_add = min([(R_max-TV_des), L_max, (T_driver-R)/2]);
            R = R + max_t_add;
            L = max_t_add;
            if ( (L + R + 0.001) < (T_driver))
                sat = uint32(1);
            end 
            T = [L;R];
            return                 
        end
    end
end

function [T, sat] = allocatePositiveTorque(L_max, R_max, T_req,...
          R_eff_L, R_eff_R, alfa, Mz_ref, GR, t, Fz_L,Fz_R )
      
    T = single(zeros(2,1));
    sat = uint32(0);
    % Desired torque vectoring torque
    TV_des = abs(alfa*Mz_ref*R_eff_L/(GR*t)) + abs(alfa*Mz_ref*R_eff_R/(GR*t));
    % Take absolute value since T_req can be negative in case of KERS
    T_driver = alfa*T_req;

    if ( Mz_ref <= 0)
        % Implies that left side should realize the TV torque,
        % since only torque >= 0 is used here.
        % Mz is defined positive counter clockwise
        L = min( [TV_des, T_driver, L_max]);
        %Max torque that can be added to both
        if L_max < abs(TV_des)
            max_t_add = single(0);
        else
            max_t_add = min([(L_max-TV_des), R_max, (T_driver-L)/2]);
        end 
        L = L + max_t_add;
        R = max_t_add;
        T = [L;R];  
        % Floats comparison
        if ( (L + R + 0.001) < (T_driver))
            sat = uint32(1);
        end
        return;
    else
        R = min( [abs(TV_des), T_driver, R_max]);
        %Max torque that can be added to both
        if R_max < abs(TV_des)
            max_t_add = single(0);
        else
            max_t_add = min([(R_max-abs(TV_des)),L_max, (T_driver-R)/2]);
        end
        R = R + max_t_add;
        L = max_t_add;
        T = [L;R];
        % Floats comparison
        if ( (L + R + 0.001) < (T_driver))
            sat = uint32(1);
        end
        return;
    end
end

function [T, sat] = allocateNegativeTorque(L_max, R_max, T_req, R_eff_L, R_eff_R, alfa, Mz_ref, GR, t, Fz_L,Fz_R )
    T = single(zeros(2,1));
    sat = uint32(0);
    % Desired torque vectoring torque
    TV_des = abs(alfa*Mz_ref*R_eff_L/(GR*t)) + abs(alfa*Mz_ref*R_eff_R/(GR*t));
    % Take absolute value since T_req can be negative in case of KERS
    T_driver = abs(alfa*T_req);
   
    if (Mz_ref + 0.0001 >= 0)
        % Positive Mz_ref requires left side (inner wheels)
        % to brake more than the outer wheels.
        L = min( [TV_des, T_driver, L_max]);
        %Max torque that can be added to both
        if L_max < abs(TV_des)
            max_t_add = single(0);
        else
            max_t_add = min([(L_max-TV_des), R_max, (T_driver-L)/2]);
        end 
        L = - (L + max_t_add);
        R = - max_t_add;
        T = [L;R];
        % Floats comparison
        if ( (abs(L) + abs(R) + 0.001) < T_driver)
            sat = uint32(1);
        end
        return;
    else
        R = min( [abs(TV_des), T_driver, R_max]);
        %Max torque that can be added to both
        if R_max < abs(TV_des)
            max_t_add = single(0);
        else
            max_t_add = min([(R_max-abs(TV_des)),L_max, (T_driver-R)/2]);
        end
        R = - (R + max_t_add);
        L = - max_t_add;
        T = [L;R];
        % Floats comparison
        if ( (abs(L) + abs(R) + 0.001) < T_driver)
            sat = uint32(1);
        end
        return;
    end
end


function [T, sat] = distOuter(L_max, R_max, T_req,...
    R_eff_L, R_eff_R, alfa, Mz_ref, GR, t, Fz_L,Fz_R )
    T = single(zeros(2,1));
    sat = uint32(0);
    % Desired torque vectoring torque
    TV_des = abs(alfa*Mz_ref*R_eff_L/(GR*t)) +...
            abs(alfa*Mz_ref*R_eff_R/(GR*t));
    % Take absolute value since T_req can be negative in case of KERS
    T_driver = abs(alfa*T_req);   
    if Fz_L >= Fz_R
        % Implies that left side should realize the TV torque
        L = min( [TV_des, T_driver, L_max]);
        %Max torque that can be added to both
        if L_max < abs(TV_des)
            max_t_add = single(0);
        else
            max_t_add = min([(L_max-TV_des), R_max, (T_driver-L)/2]);
        end 
        L = L + max_t_add;
        R = max_t_add;
        T = [L;R];
        if ( (L + R) < T_driver)
            sat = uint32(1);
        end
        return;
    elseif Fz_L < Fz_R
        R = min( [abs(TV_des), T_driver, R_max]);
        %Max torque that can be added to both
        if R_max < abs(TV_des)
            max_t_add = single(0);
        else
            max_t_add = min([(R_max-abs(TV_des)),L_max, (T_driver-R)/2]);
        end
        R = R + max_t_add;
        L = max_t_add;
        T = [L;R];
        if ( (L + R) < T_driver)
            sat = uint32(1);
        end
        return;
    end
end
